simulink model "mte484lab3"  (R2023b)
settings: Solver=ode45  StartTime=0.0  StopTime=100  FixedStep=T  MaxStep=0.01  RelTol=1e-12  AbsTol=1e-12  EnableMultiTasking=on
libraries: cstblocks x4
settings Model: Creator=cnielsen  LastModifiedBy=gs_kim
settings SolverCC: AutoScaleAbsTol=off  AlgebraicLoopSolver=TrustRegion
settings DataIOCC: SaveFormat=Array  SignalLoggingSaveFormat=ModelDataLogs  SaveOutput=off  SaveTime=off  ReturnWorkspaceOutputs=off  Refine=5
settings OptimizationCC: ExpressionDepthLimit=2147483647  LifeSpan=inf
settings DebuggingCC: UnderspecifiedInitializationDetection=Classic  MergeDetectMultiDrivingBlocksExec=none  SolverPrmCheckMsg=warning  FcnCallInpInsideContextMsg=warning  UnconnectedInputMsg=warning  UnconnectedOutputMsg=warning  UnconnectedLineMsg=warning  StateNameClashWarn=warning  SFUnexpectedBacktrackingDiag=warning  SFNoUnconditionalDefaultTransitionDiag=warning  SFExecutionAtInitializationDiag=none  ArithmeticOperatorsInVariantConditions=warning
settings HardwareCC: ProdBitPerPointer=32  ProdBitPerSizeT=32  ProdBitPerPtrDiffT=32  ProdLargestAtomicFloat=None  ProdIntDivRoundTo=Undefined  ProdEndianess=Unspecified  ProdWordSize=32  ProdHWDeviceType=32-bit Generic
settings ModelReferenceCC: PropagateSignalLabelsOutOfModel=off
settings SFSimCC: SimUseLocalCustomCode=off  CustomCodeUndefinedFunction=UseInterfaceOnly
settings RTWCC: RTWUseLocalCustomCode=off
settings CodeAppCC: StateflowObjectComments=on
settings GRTTargetCC: TargetLangStandard=C89/C90 (ANSI)  CombineOutputUpdateFcns=off  GRTInterface=on
settings ConfigComp: CovMetricSettings=dw  CovSaveCumulativeToWorkspaceVar=on  CovSaveSingleToWorkspaceVar=on  CovExternalEMLEnable=off

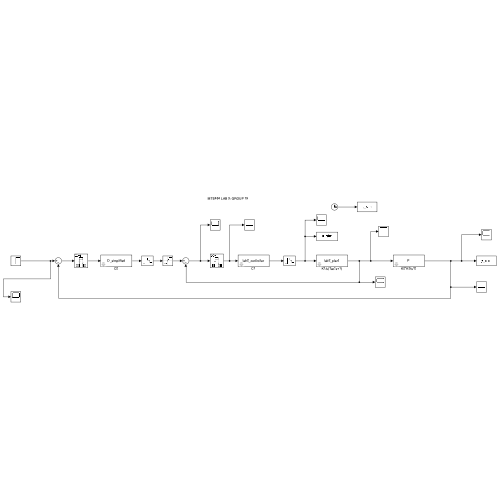
[thumbnail: Simulink's stored preview of the top-level diagram]
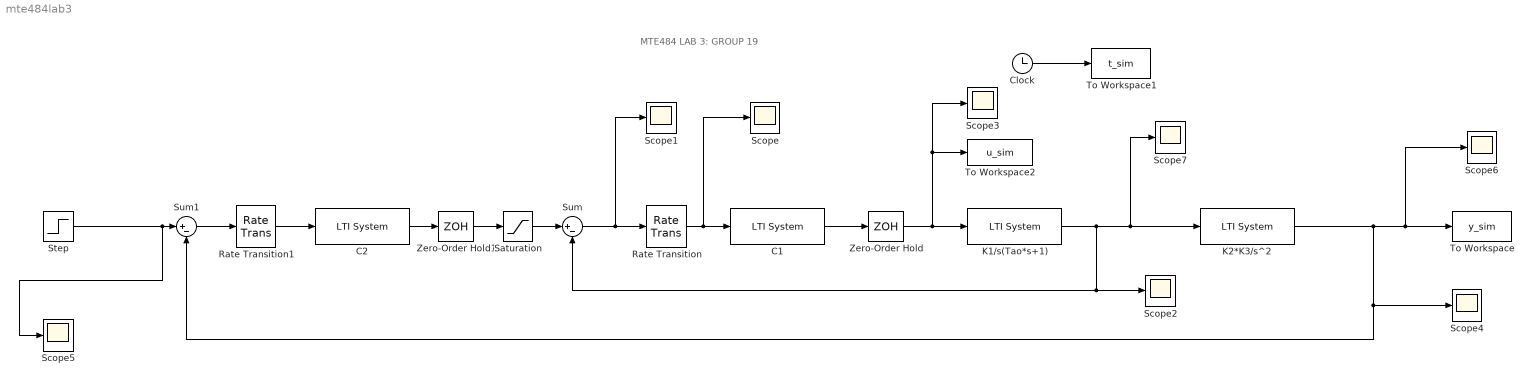
== system mte484lab3 ==
  note: MTE484 LAB 3: GROUP 19
  C1 : cstblocks/LTI System  sys=lab2_controller  IC=[]  PadeOrder=0
  C2 : cstblocks/LTI System  sys=D_simplified  IC=[]  PadeOrder=0
  Clock : Clock
  K1/s(Tao*s+1) : cstblocks/LTI System  sys=lab2_plant  IC=[]  PadeOrder=0
  K2*K3/s^2 : cstblocks/LTI System  sys=P  IC=[]  PadeOrder=0
  Rate Transition : RateTransition  OutPortSampleTime=0.009
  Rate Transition1 : RateTransition  OutPortSampleTime=0.45
  Saturation : Saturate  UpperLimit=0.7  LowerLimit=-0.7
  Scope{,1..7} (8 alike) : Scope
  Step : Step  Time=0  Before=0.0  After=0.15
  Sum : Sum  Inputs=|+-
  Sum1 : Sum  Inputs=|+-
  To Workspace : ToWorkspace  VariableName=y_sim  SampleTime=-1
  To Workspace1 : ToWorkspace  VariableName=t_sim  SampleTime=-1
  To Workspace2 : ToWorkspace  VariableName=u_sim
  Zero-Order Hold : ZeroOrderHold  SampleTime=0.009
  Zero-Order Hold1 : ZeroOrderHold  SampleTime=0.45
  wires:
  Clock/1 -> To Workspace1/1
  C1/1 -> Zero-Order Hold/1
  Sum/1 -> Rate Transition/1, Scope1/1
  Zero-Order Hold/1 -> K1/s(Tao*s+1)/1, To Workspace2/1, Scope3/1
  Rate Transition/1 -> C1/1, Scope/1
  C2/1 -> Zero-Order Hold1/1
  Rate Transition1/1 -> C2/1
  K1/s(Tao*s+1)/1 -> Scope7/1, K2*K3/s^2/1, Sum/2, Scope2/1
  K2*K3/s^2/1 -> Sum1/2, Scope4/1, Scope6/1, To Workspace/1
  Step/1 -> Scope5/1, Sum1/1
  Sum1/1 -> Rate Transition1/1
  Zero-Order Hold1/1 -> Saturation/1
  Saturation/1 -> Sum/1
